simulink model "untitled"  (R2023a)
settings: Solver=VariableStepAuto  StartTime=0.0  StopTime=10.0  RelTol=1e-3
values from neighbouring files (symbols this model uses):
  R = log([7, 10, 20, 30, 40, 50])    [exp7.m]    (also in exp7a.m = [7, 10, 20, 30, 40, 50])
undefined symbols (not defined in the file or in its folder): A
settings Model: Creator=FC  LastModifiedBy=FC

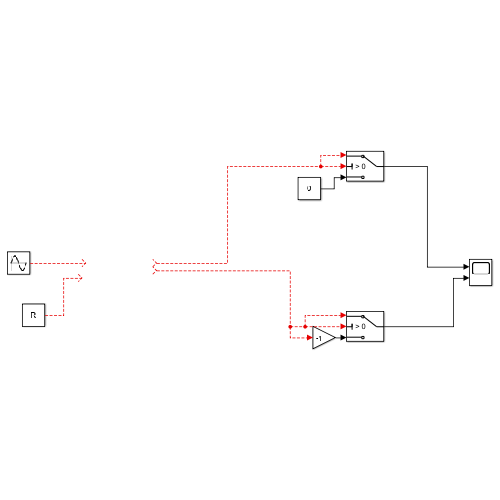
[thumbnail: Simulink's stored preview of the top-level diagram]
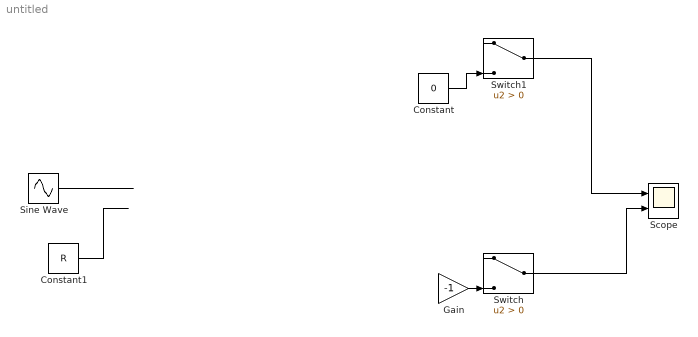
== system untitled ==
  Constant : Constant  Value=0
  Constant1 : Constant  Value=R
  Gain : Gain  Gain=-1
  Scope : Scope  NumInputPorts=2
  Sine Wave : Sin  Amplitude=A  SampleTime=0
  Switch : Switch  Criteria=u2 > Threshold  SaturateOnIntegerOverflow=off  InputSameDT=off
  Switch1 : Switch  Criteria=u2 > Threshold  SaturateOnIntegerOverflow=off  InputSameDT=off
  wires:
  Gain/1 -> Switch/3
  Constant/1 -> Switch1/3
  Sine Wave/1 -> ?
  ? -> Switch1/1, Switch1/2
  ? -> Gain/1, Switch/1, Switch/2
  Switch/1 -> Scope/2
  Switch1/1 -> Scope/1
  Constant1/1 -> ?
